simulink model "quad_6D0F_ASMC"  (R2023a)
settings: Solver=ode1  StartTime=0.0  StopTime=10.0  FixedStep=0.01  RelTol=1e-3
libraries: matrix_library x1, robotcorelib x1
settings Model: Creator=Adan Daniel  LastModifiedBy=Adan Daniel

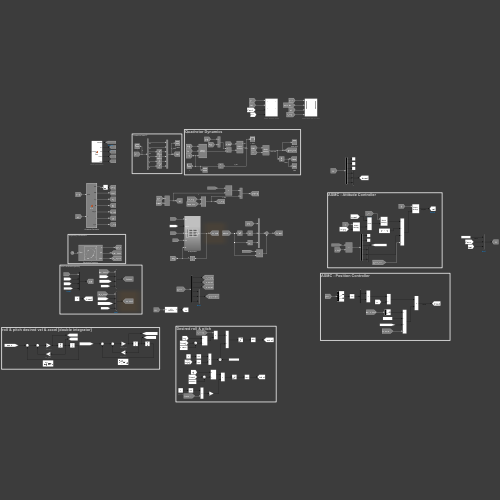
[thumbnail: Simulink's stored preview of the top-level diagram]
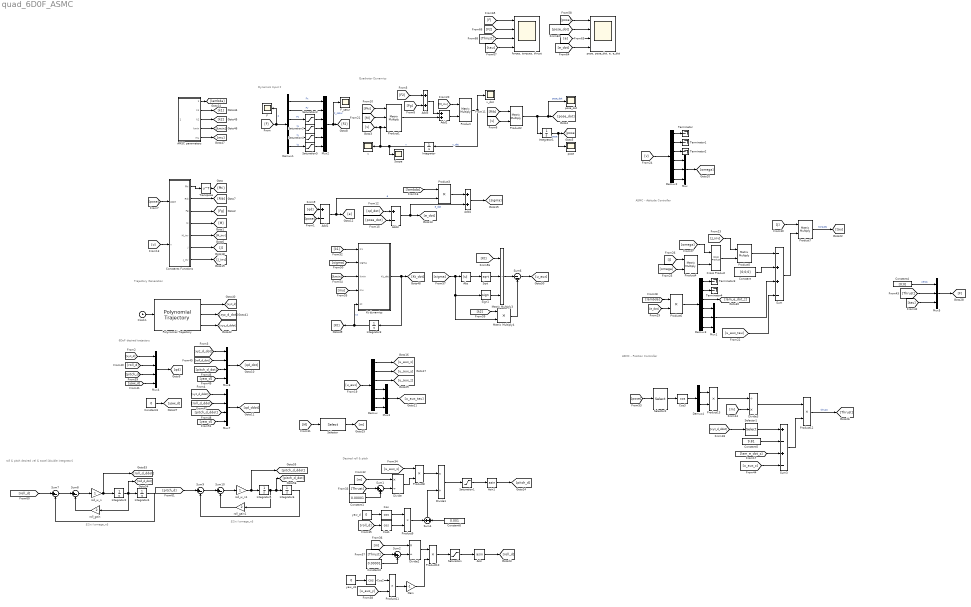
== system quad_6D0F_ASMC ==
  note: roll & pitch desired vel & accel [double integrator]
  note: Desired roll & pitch
  note: ASMC - Attitude Controller
  note: Quadrotor Dynamics
  note: Trajectory Generation
  note: Dynamics Input F
  note: $2\xi \omega_n$
  note: $2\xi \omega_n$
  note: 6DoF desired trajectory
  note: ASMC - Position Controller
  AMSC parameters : MATLAB Function  TreatAsAtomicUnit=on
  Abs : Abs  SaturateOnIntegerOverflow=off
  Add1 : Sum  Inputs=+-
  Add2 : Sum
  Add3 : Sum  Inputs=+-
  Add4 : Sum
  Add5 : Sum
  Asin : Trigonometry  Operator=asin
  Asin1 : Trigonometry  Operator=asin
  Clock1 : Clock
  Constant : Constant  Value=[0;0;0]
  Constant1 : Constant  Value=0.00001
  Constant2 : Constant  Value=0.00001
  Constant3 : Constant  Value=0
  Constant4 : Constant  Value=[0;0]
  Constant5 : Constant  Value=9.81
  Constant6 : Constant  Value=0.001
  Constants Functions : MATLAB Function  TreatAsAtomicUnit=on
  Cos{,1..3} (4 alike) : Trigonometry  Operator=cos
  Cross Product : matrix_library/Cross Product
  Demux{,1..3} (4 alike) : Demux  Outputs=6
  Demux4 : Demux  Outputs=2
  Divide : Product  Inputs=*/
  Divide1 : Product  Inputs=*/
  Divide2 : Product  Inputs=*/
  Divide3 : Product  Inputs=/*
  F : Scope
  F_satur : Scope
  Gain : Gain  Gain=-1
  Integrator : Integrator  InitialCondition=[0; 0; 0; 0; 0; 0]
  Integrator1 : Integrator  InitialCondition=[0; 0; 0; 0; 0; 0]
  Integrator{2,4..6} (4 alike) : Integrator
  Integrator3 : Integrator  InitialCondition=[0; 0; 0; 0; 0; 0]
  Kt dynamics : Subsystem
  Matrix Multiply3 : Product  Inputs=3
  Matrix Multiply4 : Product
  Mux{,1,3,5} (4 alike) : Mux  Inputs=3
  Mux2 : Mux  Inputs=6
  Mux4 : Mux
  Mux6 : Mux
  Mux7 : Mux
  Polynomial Trajectory : robotcorelib/Polynomial Trajectory  WaypointSource=Internal  Waypoints=[0, 0, 0, 0, 0, 0; 0, 0, 0, 0, 0, 0; 0, 0, 0, 0, 0, 0]  TimePoints=[ 0, 12, 24, 35, 48, 60]  TimeInterval=[ 1, 4 ]  Method=Cubic Polynomial  ParameterSource=Internal  VelocityBoundaryCondition=zeros( 3, 6)  AccelerationBoundaryCondition=zeros( 2, 5 )  SimulateUsing=Interpreted execution
  Product{,2,4..5,7} (5 alike) : Product  Multiplication=Matrix(*)
  Product1 : Product  Inputs=3  Multiplication=Matrix(*)
  Product{3,6,8..13} (8 alike) : Product
  Saturation : Saturate  UpperLimit=1  LowerLimit=-1
  Saturation1 : Saturate  UpperLimit=1  LowerLimit=-1
  Saturation2 : Saturate  UpperLimit=5.8*6  LowerLimit=0
  Saturation3 : Saturate
  Saturation4 : Saturate
  Saturation5 : Saturate
  Scope : Scope
  Selector : Selector  NumberOfDimensions=2  InputPortWidth=3  IndexOptions=Index vector (dialog),Index vector (dialog)  Indices=1,1  OutputSizes=1,1
  Selector1 : Selector  InputPortWidth=3  IndexOptions=Index vector (dialog)  Indices=3  OutputSizes=1
  Selector2 : Selector  InputPortWidth=6  IndexOptions=Index vector (dialog)  Indices=[4 5]  OutputSizes=1
  Sign1 : Signum
  Sqrt : Sqrt
  Sum : Sum  Inputs=-++-
  Sum1 : Sum  Inputs=|++
  Sum{7..10} (4 alike) : Sum  Inputs=|+-
  Sum2 : Sum  Inputs=|++
  Sum3 : Sum  Inputs=+-+-
  Sum4 : Sum
  Sum6 : Sum  Inputs=|--
  Terminator{,1..4} (5 alike) : Terminator
  Transpose : Math  Operator=transpose
  "forces, torques, thrust" : Scope  NumInputPorts=4
  pose : Scope
  "pose, pose_dot, e, e_dot" : Scope  NumInputPorts=4
  pose_dot : Scope
  roll_gain : Gain  Gain=2
  roll_gain1 : Gain  Gain=2
  roll_w_n : Gain
  roll_w_n1 : Gain
  v : Scope
  v_dot : Scope
  yaw_d : Constant  Value=0
  yaw_d1 : Constant  Value=0
  wires:
  [v] -> Product2/2
  Product2/1 -> Integrator1/1, pose_dot/1, [pose_dot]  "pose_dot"
  Product/1 -> v_dot/1, Integrator/1  "v_dot"
  Integrator1/1 -> pose/1, [pose]  "pose"
  Integrator/1 -> Scope/1, v/1, [v], Product1/3  "v"
  Add5/1 -> Add2/1
  [M] -> Product1/2
  [Fg] -> Add5/2
  Add2/1 -> Product/2
  [Rib] -> Product2/1
  [Phi] -> Product1/1
  Product1/1 -> Add2/2
  [F2] -> Add5/1
  [M_inv] -> Product/1
  [pose] -> Constants Functions/1(pose)
  [v] -> Constants Functions/2(v)
  Constants Functions/1(Phi) -> Transpose/1
  Constants Functions/4(M) -> [M]
  Constants Functions/3(Fg) -> [Fg]
  Constants Functions/5(M_inv) -> [M_inv]
  Constants Functions/2(Rib) -> [Rib]
  Transpose/1 -> [Phi]
  Clock1/1 -> Polynomial Trajectory/1
  Saturation5/1 -> Mux2/6
  Demux1/5 -> Saturation4/1  "ty"
  Saturation3/1 -> Mux2/4
  Saturation2/1 -> Mux2/3
  Demux1/1 -> Mux2/1  "Fx"
  Demux1/2 -> Mux2/2  "Fy"
  Mux2/1 -> F_satur/1, [F2]  "F_satur"
  [F] -> F/1, Demux1/1  "F"
  Saturation4/1 -> Mux2/5
  Demux1/6 -> Saturation5/1  "tz"
  Demux1/4 -> Saturation3/1  "tx"
  Demux1/3 -> Saturation2/1  "Fz"
  AMSC parameters/5(mu) -> [mu]
  AMSC parameters/2(k1) -> [k1]
  AMSC parameters/3(k2) -> [k2]
  AMSC parameters/4(kmin) -> [kmin]
  Polynomial Trajectory/1 -> [xyz_d]
  Polynomial Trajectory/2 -> [xyz_d_dot]
  Polynomial Trajectory/3 -> [xyz_d_ddot]
  [qd] -> Add1/1
  [pose] -> Add1/2
  [qd_dot] -> Add3/1
  AMSC parameters/1(lambda) -> [lambda]
  [lambda] -> Product3/1
  Add1/1 -> Product3/2, [e]  "e"
  Product3/1 -> Add4/1
  Add3/1 -> Add4/2, [e_dot]  "e_dot"
  Add4/1 -> [sigma]
  Abs/1 -> Sqrt/1
  Integrator3/1 -> [Kt], Kt dynamics/5(Kt)  "Kt"
  [sigma] -> Matrix Multiply4/2, Sign1/1, Abs/1
  Sign1/1 -> Matrix Multiply3/3
  Matrix Multiply4/1 -> Sum6/2
  [mu] -> Kt dynamics/4(mu)
  Sqrt/1 -> Matrix Multiply3/2
  [k2] -> Matrix Multiply4/1
  [sigma] -> Kt dynamics/2(sigma)
  [k1] -> Kt dynamics/1(K1)
  [Kt] -> Matrix Multiply3/1
  [kmin] -> Kt dynamics/3(Kmin)
  Matrix Multiply3/1 -> Sum6/1
  Kt dynamics/1(Kt_dot) -> Integrator3/1, [Kt_dot]
  Sum6/1 -> [u_aux]
  [u_aux] -> Demux/1
  Demux/1 -> [u_aux_x]
  Demux/2 -> [u_aux_y]
  Constants Functions/7(J_inv) -> [J_inv]
  Constants Functions/6(J) -> [J]
  [v] -> Demux2/1
  Demux2/4 -> Mux/1
  Demux2/6 -> Mux/3
  Demux2/5 -> Mux/2
  Mux/1 -> [omega]
  [J] -> Product4/1
  [omega] -> Product4/2
  Product4/1 -> Cross Product/2
  [omega] -> Cross Product/1
  Cross Product/1 -> Product5/2
  [J_inv] -> Product5/1
  [lambda] -> Product6/1
  [e_dot] -> Product6/2
  Mux1/1 -> Sum/3
  Demux3/4 -> Mux1/1
  Demux3/6 -> Mux1/3
  Demux3/5 -> Mux1/2
  Product6/1 -> Demux3/1
  Mux3/1 -> [u_aux_tau]
  Demux/4 -> Mux3/1
  Demux/6 -> Mux3/3
  Demux/5 -> Mux3/2
  Product5/1 -> Sum/1
  Constant/1 -> Sum/2
  [u_aux_tau] -> Sum/4
  [J] -> Product7/1
  Sum/1 -> Product7/2
  Product7/1 -> [tau]  "torques"
  [M] -> Selector/1
  Selector/1 -> [m]
  [pose_dot] -> Add3/2
  Constant3/1 -> [yaw_d]
  [yaw_d] -> Mux4/4
  [pitch_d] -> Mux4/3
  [roll_d] -> Mux4/2
  [xyz_d] -> Mux4/1
  Mux4/1 -> [qd]
  Demux2/1 -> Terminator/1
  Demux2/2 -> Terminator1/1
  Demux2/3 -> Terminator2/1
  Demux3/2 -> Terminator4/1
  Demux3/1 -> Terminator3/1
  Demux3/3 -> [lam_e_dot_z]
  Constant4/1 -> Mux5/1  "zeros"
  [Thrust] -> Mux5/2
  [tau] -> Mux5/3
  Mux5/1 -> [F]
  Demux/3 -> [u_aux_z]
  Divide1/1 -> Saturation1/1
  [u_aux_y] -> Product11/2
  Cos1/1 -> Product9/2
  [m] -> Divide2/1
  Sum1/1 -> Divide/2
  Gain/1 -> Product10/2
  [Thrust] -> Sum2/1
  yaw_d1/1 -> Cos2/1
  Constant1/1 -> Sum1/2
  Product11/1 -> Gain/1
  Cos/1 -> Product9/1
  Product10/1 -> Saturation/1
  Constant2/1 -> Sum2/2
  [roll_d] -> Cos1/1
  Divide2/1 -> Product10/1
  Divide/1 -> Product8/2
  Sum2/1 -> Divide2/2
  [u_aux_x] -> Product8/1
  Cos2/1 -> Product11/1
  Asin1/1 -> [pitch_d]
  [Thrust] -> Sum1/1
  Saturation/1 -> Asin/1
  Saturation1/1 -> Asin1/1
  yaw_d/1 -> Cos/1
  Product8/1 -> Divide1/1
  [m] -> Divide/1
  Asin/1 -> [roll_d]
  Sum7/1 -> Sum8/1
  [roll_d] -> Sum7/1
  Integrator2/1 -> [roll_d_dot], Integrator4/1, roll_gain/1
  roll_gain/1 -> Sum8/2
  Integrator6/1 -> Sum9/2
  Sum9/1 -> Sum10/1
  Sum8/1 -> roll_w_n/1
  Integrator4/1 -> Sum7/2
  Integrator5/1 -> roll_gain1/1, [pitch_d_dot], Integrator6/1
  roll_w_n/1 -> [roll_d_ddot], Integrator2/1
  roll_w_n1/1 -> [pitch_d_ddot], Integrator5/1
  roll_gain1/1 -> Sum10/2
  [pitch_d] -> Sum9/1
  Sum10/1 -> roll_w_n1/1
  [yaw_d] -> Mux6/4
  [roll_d_dot] -> Mux6/2
  [xyz_d_dot] -> Mux6/1
  [pitch_d_dot] -> Mux6/3
  Mux6/1 -> [qd_dot]
  [yaw_d] -> Mux7/4
  [roll_d_ddot] -> Mux7/2
  [xyz_d_ddot] -> Mux7/1
  [pitch_d_ddot] -> Mux7/3
  Mux7/1 -> [qd_ddot]
  [u_aux_z] -> Sum3/4
  [lam_e_dot_z] -> Sum3/3
  Constant5/1 -> Sum3/2
  Selector1/1 -> Sum3/1
  [xyz_d_ddot] -> Selector1/1
  [pose] -> Selector2/1
  Selector2/1 -> Cos3/1
  Cos3/1 -> Demux4/1
  Demux4/1 -> Product13/1
  Demux4/2 -> Product13/2
  [m] -> Divide3/2
  Sum3/1 -> Product12/2
  Divide3/1 -> Product12/1
  Product13/1 -> Divide3/1
  Product12/1 -> [Thrust]  "thrust"
  [pose] -> "pose, pose_dot, e, e_dot"/1
  [e_dot] -> "pose, pose_dot, e, e_dot"/4
  [e] -> "pose, pose_dot, e, e_dot"/3
  [pose_dot] -> "pose, pose_dot, e, e_dot"/2
  [tau] -> "forces, torques, thrust"/4
  [F2] -> "forces, torques, thrust"/2
  [F] -> "forces, torques, thrust"/1
  [Thrust] -> "forces, torques, thrust"/3
  Product9/1 -> Sum4/1
  Sum4/1 -> Divide1/2
  Constant6/1 -> Sum4/2

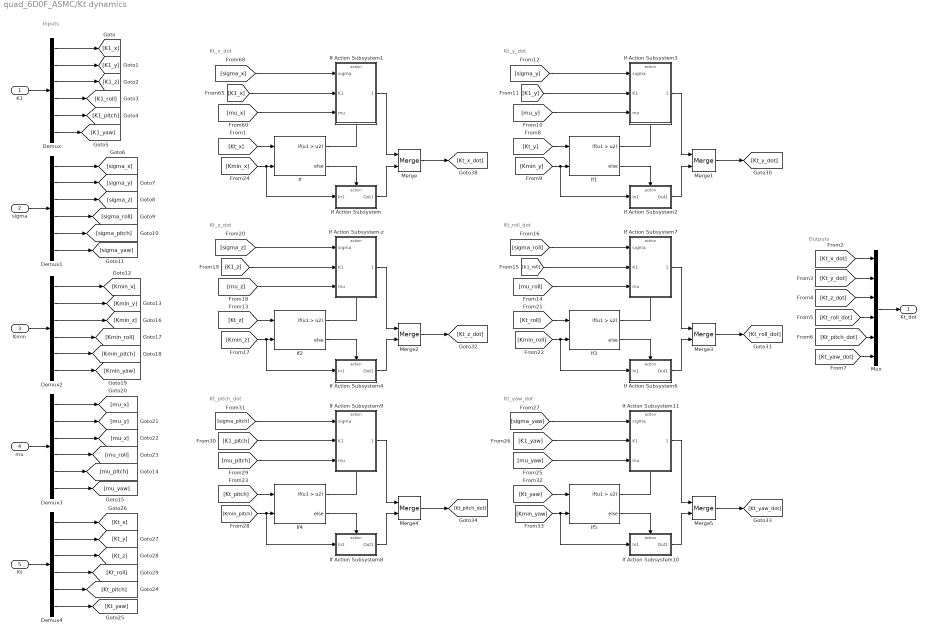
== system quad_6D0F_ASMC/Kt dynamics ==
  note: Outputs
  note: Inputs
  note: Kt_x_dot
  note: Kt_y_dot
  note: Kt_z_dot
  note: Kt_roll_dot
  note: Kt_pitch_dot
  note: Kt_yaw_dot
  K1 : Inport
  sigma : Inport  Port=2
  Kmin : Inport  Port=3
  mu : Inport  Port=4
  Kt : Inport  Port=5
  Demux{,1..4} (5 alike) : Demux  Outputs=6
  If{,1..5} (6 alike) : If  NumInputs=2  IfExpression=u1 > u2
  If Action Subsystem : Subsystem  TreatAsAtomicUnit=on
  If Action Subsystem-z : Subsystem  TreatAsAtomicUnit=on
  If Action Subsystem1 : Subsystem  TreatAsAtomicUnit=on
  If Action Subsystem10 : Subsystem  TreatAsAtomicUnit=on
  If Action Subsystem11 : Subsystem  TreatAsAtomicUnit=on
  If Action Subsystem2 : Subsystem  TreatAsAtomicUnit=on
  If Action Subsystem3 : Subsystem  TreatAsAtomicUnit=on
  If Action Subsystem4 : Subsystem  TreatAsAtomicUnit=on
  If Action Subsystem6 : Subsystem  TreatAsAtomicUnit=on
  If Action Subsystem7 : Subsystem  TreatAsAtomicUnit=on
  If Action Subsystem8 : Subsystem  TreatAsAtomicUnit=on
  If Action Subsystem9 : Subsystem  TreatAsAtomicUnit=on
  Merge{,1..5} (6 alike) : Merge
  Mux : Mux  Inputs=6
  Kt_dot : Outport
  wires:
  [Kt_x] -> If/1
  [sigma_x] -> If Action Subsystem1/1(sigma)
  If/1 -> If Action Subsystem1/Action
  [K1_x] -> If Action Subsystem1/2(K1)
  If Action Subsystem1/1(Kt_x_dot) -> Merge/1
  If Action Subsystem/1(Out1) -> Merge/2
  If/2 -> If Action Subsystem/Action
  Merge/1 -> [Kt_x_dot]
  [Kmin_x] -> If Action Subsystem/1(In1), If/2
  [mu_x] -> If Action Subsystem1/3(mu)
  Merge1/1 -> [Kt_y_dot]
  If1/2 -> If Action Subsystem2/Action
  If Action Subsystem2/1(Out1) -> Merge1/2
  If Action Subsystem3/1(Kt_x_dot) -> Merge1/1
  [Kt_y] -> If1/1
  [K1_y] -> If Action Subsystem3/2(K1)
  [mu_y] -> If Action Subsystem3/3(mu)
  [Kmin_y] -> If Action Subsystem2/1(In1), If1/2
  [sigma_y] -> If Action Subsystem3/1(sigma)
  Merge2/1 -> [Kt_z_dot]
  If Action Subsystem-z/1(Kt_z_dot) -> Merge2/1
  [sigma_z] -> If Action Subsystem-z/1(sigma)
  [Kt_z] -> If2/1
  [mu_z] -> If Action Subsystem-z/3(mu)
  [Kmin_z] -> If Action Subsystem4/1(In1), If2/2
  If3/2 -> If Action Subsystem6/Action
  If Action Subsystem7/1(Kt_x_dot) -> Merge3/1
  Merge3/1 -> [Kt_roll_dot]
  If3/1 -> If Action Subsystem7/Action
  [Kmin_roll] -> If Action Subsystem6/1(In1), If3/2
  If2/2 -> If Action Subsystem4/Action
  [sigma_roll] -> If Action Subsystem7/1(sigma)
  If2/1 -> If Action Subsystem-z/Action
  [K1_roll] -> If Action Subsystem7/2(K1)
  If Action Subsystem6/1(Out1) -> Merge3/2
  [mu_roll] -> If Action Subsystem7/3(mu)
  If Action Subsystem4/1(Out1) -> Merge2/2
  [Kt_roll] -> If3/1
  [K1_z] -> If Action Subsystem-z/2(K1)
  Merge4/1 -> [Kt_pitch_dot]
  If Action Subsystem9/1(Kt_x_dot) -> Merge4/1
  [sigma_pitch] -> If Action Subsystem9/1(sigma)
  [Kt_pitch] -> If4/1
  [mu_pitch] -> If Action Subsystem9/3(mu)
  [Kmin_pitch] -> If Action Subsystem8/1(In1), If4/2
  If5/2 -> If Action Subsystem10/Action
  If Action Subsystem11/1(Kt_x_dot) -> Merge5/1
  Merge5/1 -> [Kt_yaw_dot]
  If5/1 -> If Action Subsystem11/Action
  [Kmin_yaw] -> If Action Subsystem10/1(In1), If5/2
  If4/2 -> If Action Subsystem8/Action
  [sigma_yaw] -> If Action Subsystem11/1(sigma)
  If4/1 -> If Action Subsystem9/Action
  [K1_yaw] -> If Action Subsystem11/2(K1)
  If Action Subsystem10/1(Out1) -> Merge5/2
  [mu_yaw] -> If Action Subsystem11/3(mu)
  If Action Subsystem8/1(Out1) -> Merge4/2
  [Kt_yaw] -> If5/1
  [K1_pitch] -> If Action Subsystem9/2(K1)
  If1/1 -> If Action Subsystem3/Action
  Demux4/6 -> [Kt_yaw]
  Demux4/1 -> [Kt_x]
  Demux1/5 -> [sigma_pitch]
  Demux1/3 -> [sigma_z]
  Demux1/1 -> [sigma_x]
  Demux1/2 -> [sigma_y]
  Kt/1 -> Demux4/1
  Demux4/4 -> [Kt_roll]
  sigma/1 -> Demux1/1
  Demux3/4 -> [mu_roll]
  Demux2/4 -> [Kmin_roll]
  Demux3/1 -> [mu_x]
  Demux2/3 -> [Kmin_z]
  Demux3/3 -> [mu_z]
  mu/1 -> Demux3/1
  Demux3/6 -> [mu_yaw]
  Demux3/5 -> [mu_pitch]
  Demux2/5 -> [Kmin_pitch]
  Demux3/2 -> [mu_y]
  Demux2/6 -> [Kmin_yaw]
  Demux2/1 -> [Kmin_x]
  Demux2/2 -> [Kmin_y]
  Demux/4 -> [K1_roll]
  Demux1/4 -> [sigma_roll]
  Demux4/5 -> [Kt_pitch]
  Demux4/2 -> [Kt_y]
  Demux4/3 -> [Kt_z]
  Demux/1 -> [K1_x]
  K1/1 -> Demux/1
  Demux/6 -> [K1_yaw]
  Demux/5 -> [K1_pitch]
  Demux1/6 -> [sigma_yaw]
  Demux/2 -> [K1_y]
  Kmin/1 -> Demux2/1
  Demux/3 -> [K1_z]
  Mux/1 -> Kt_dot/1
  [Kt_z_dot] -> Mux/3
  [Kt_yaw_dot] -> Mux/6
  [Kt_pitch_dot] -> Mux/5
  [Kt_x_dot] -> Mux/1
  [Kt_y_dot] -> Mux/2
  [Kt_roll_dot] -> Mux/4

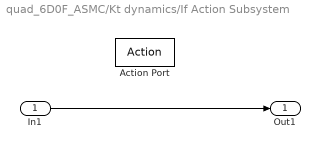
== system quad_6D0F_ASMC/Kt dynamics/If Action Subsystem ==
  In1 : Inport
  Action Port : ActionPort  ActionPortLabel=else
  Out1 : Outport
  wires:
  In1/1 -> Out1/1

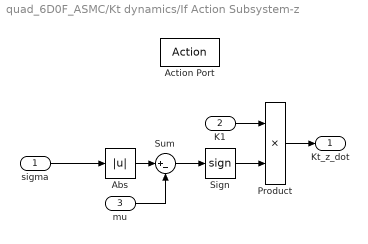
== system quad_6D0F_ASMC/Kt dynamics/If Action Subsystem-z ==
  sigma : Inport
  K1 : Inport  Port=2
  mu : Inport  Port=3
  Action Port : ActionPort  ActionPortLabel=if(u1 > u2)
  Abs : Abs  SaturateOnIntegerOverflow=off
  Product : Product
  Sign : Signum
  Sum : Sum  Inputs=|+-
  Kt_z_dot : Outport
  wires:
  sigma/1 -> Abs/1
  Abs/1 -> Sum/1
  mu/1 -> Sum/2
  Sum/1 -> Sign/1
  Product/1 -> Kt_z_dot/1
  Sign/1 -> Product/2
  K1/1 -> Product/1

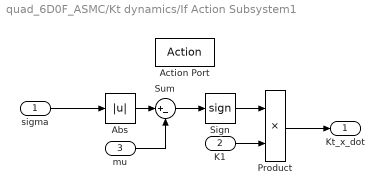
== system quad_6D0F_ASMC/Kt dynamics/If Action Subsystem1 ==
  sigma : Inport
  K1 : Inport  Port=2
  mu : Inport  Port=3
  Action Port : ActionPort  ActionPortLabel=if(u1 > u2)
  Abs : Abs  SaturateOnIntegerOverflow=off
  Product : Product
  Sign : Signum
  Sum : Sum  Inputs=|+-
  Kt_x_dot : Outport
  wires:
  sigma/1 -> Abs/1
  Abs/1 -> Sum/1
  mu/1 -> Sum/2
  Sum/1 -> Sign/1
  Sign/1 -> Product/1
  K1/1 -> Product/2
  Product/1 -> Kt_x_dot/1

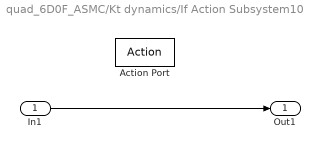
== system quad_6D0F_ASMC/Kt dynamics/If Action Subsystem10 ==
  In1 : Inport
  Action Port : ActionPort  ActionPortLabel=else
  Out1 : Outport
  wires:
  In1/1 -> Out1/1

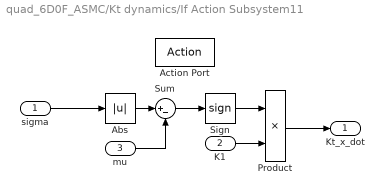
== system quad_6D0F_ASMC/Kt dynamics/If Action Subsystem11 ==
  sigma : Inport
  K1 : Inport  Port=2
  mu : Inport  Port=3
  Action Port : ActionPort  ActionPortLabel=if(u1 > u2)
  Abs : Abs  SaturateOnIntegerOverflow=off
  Product : Product
  Sign : Signum
  Sum : Sum  Inputs=|+-
  Kt_x_dot : Outport
  wires:
  sigma/1 -> Abs/1
  Abs/1 -> Sum/1
  mu/1 -> Sum/2
  Sum/1 -> Sign/1
  Sign/1 -> Product/1
  K1/1 -> Product/2
  Product/1 -> Kt_x_dot/1

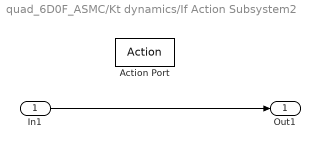
== system quad_6D0F_ASMC/Kt dynamics/If Action Subsystem2 ==
  In1 : Inport
  Action Port : ActionPort  ActionPortLabel=else
  Out1 : Outport
  wires:
  In1/1 -> Out1/1

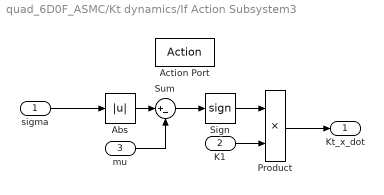
== system quad_6D0F_ASMC/Kt dynamics/If Action Subsystem3 ==
  sigma : Inport
  K1 : Inport  Port=2
  mu : Inport  Port=3
  Action Port : ActionPort  ActionPortLabel=if(u1 > u2)
  Abs : Abs  SaturateOnIntegerOverflow=off
  Product : Product
  Sign : Signum
  Sum : Sum  Inputs=|+-
  Kt_x_dot : Outport
  wires:
  sigma/1 -> Abs/1
  Abs/1 -> Sum/1
  mu/1 -> Sum/2
  Sum/1 -> Sign/1
  Sign/1 -> Product/1
  K1/1 -> Product/2
  Product/1 -> Kt_x_dot/1

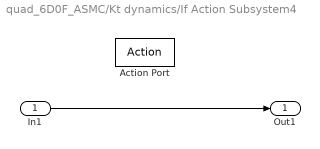
== system quad_6D0F_ASMC/Kt dynamics/If Action Subsystem4 ==
  In1 : Inport
  Action Port : ActionPort  ActionPortLabel=else
  Out1 : Outport
  wires:
  In1/1 -> Out1/1

== system quad_6D0F_ASMC/Kt dynamics/If Action Subsystem6 ==
  In1 : Inport
  Action Port : ActionPort  ActionPortLabel=else
  Out1 : Outport
  wires:
  In1/1 -> Out1/1

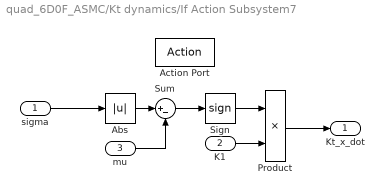
== system quad_6D0F_ASMC/Kt dynamics/If Action Subsystem7 ==
  sigma : Inport
  K1 : Inport  Port=2
  mu : Inport  Port=3
  Action Port : ActionPort  ActionPortLabel=if(u1 > u2)
  Abs : Abs  SaturateOnIntegerOverflow=off
  Product : Product
  Sign : Signum
  Sum : Sum  Inputs=|+-
  Kt_x_dot : Outport
  wires:
  sigma/1 -> Abs/1
  Abs/1 -> Sum/1
  mu/1 -> Sum/2
  Sum/1 -> Sign/1
  Sign/1 -> Product/1
  K1/1 -> Product/2
  Product/1 -> Kt_x_dot/1

== system quad_6D0F_ASMC/Kt dynamics/If Action Subsystem8 ==
  In1 : Inport
  Action Port : ActionPort  ActionPortLabel=else
  Out1 : Outport
  wires:
  In1/1 -> Out1/1

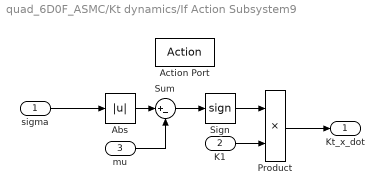
== system quad_6D0F_ASMC/Kt dynamics/If Action Subsystem9 ==
  sigma : Inport
  K1 : Inport  Port=2
  mu : Inport  Port=3
  Action Port : ActionPort  ActionPortLabel=if(u1 > u2)
  Abs : Abs  SaturateOnIntegerOverflow=off
  Product : Product
  Sign : Signum
  Sum : Sum  Inputs=|+-
  Kt_x_dot : Outport
  wires:
  sigma/1 -> Abs/1
  Abs/1 -> Sum/1
  mu/1 -> Sum/2
  Sum/1 -> Sign/1
  Sign/1 -> Product/1
  K1/1 -> Product/2
  Product/1 -> Kt_x_dot/1

== matlab function quad_6D0F_ASMC/AMSC parameters ==
  data: lambda output; unused input; k1 output; k2 output; kmin output; mu output
function [lambda, k1, k2, kmin, mu]= fcn(~)

lambda = [1; 1; 1; 1; 1; 1];

k1 = [1; 1; 1; 1; 1; 1];

k2 = [1; 1; 1; 1; 1; 1];

kmin = [1; 1; 1; 1; 1; 1];

mu = [0.01; 0.01; 0.01; 0.01; 0.01; 0.01];

== matlab function quad_6D0F_ASMC/Constants Functions ==
  data: Phi output; Rib output; Fg output; pose input; M output; M_inv output; v input; J output; J_inv output
function [Phi, Rib, Fg, M, M_inv, J, J_inv]   = fcn(pose, v)

%% System constants
m = 2; %5 mass 2.2 kg
l = 0.25; % m
g = 9.81; % gravity
Jxx =  0.0411; % kg m²
Jyy = 0.0478; % kg m²
Jzz = 0.0599; % kg m²
kT = 3.4e-5;
kQ = 3.4e-6;
%% Phi vector 6d

uu = v(1);
vv = v(2);
ww = v(3);
pp = v(4);
qq = v(5);
rr = v(6);


Phi = [0, -rr, qq, 0, -ww, vv;
        rr, 0, -pp , ww, 0, -uu;
        -qq, pp, 0,  -vv, uu, 0;
        0, 0, 0, 0, -rr, qq; 
        0, 0, 0, rr, 0, -pp;
        0, 0, 0, -qq, pp, 0];
%% Fg and Rib calculation

roll = pose(4);
pitch = pose(5);
yaw = pose(6);


Rib = [cos(yaw)*cos(pitch), -cos(roll)*sin(yaw) + cos(yaw)*sin(roll)*sin(pitch), sin(roll)*sin(yaw) + cos(roll)*cos(yaw)*sin(pitch), 0, 0, 0;
       cos(pitch)*sin(yaw), cos(roll)*cos(yaw) + sin(yaw)*sin(pitch)*sin(roll), -cos(yaw)*sin(roll) + sin(yaw)*sin(pitch)*cos(roll), 0, 0, 0;
       -sin(pitch), cos(pitch)*sin(roll), cos(pitch)*cos(roll), 0, 0, 0;
       0, 0, 0, 1, sin(roll)*tan(pitch), cos(roll)*tan(pitch);
       0, 0, 0, 0, cos(roll), -sin(roll);
       0, 0, 0, 0, sin(roll)/cos(pitch), cos(roll)/cos(pitch)];

Fg = [m*g*sin(pitch);
      -m*g*cos(pitch)*sin(roll);
      -m*g*cos(pitch)*cos(roll);
      0;
      0;
      0];

%% M matrix

M = [m, 0, 0, 0, 0, 0;
    0, m, 0, 0, 0, 0;
    0, 0, m, 0, 0, 0;
    0, 0, 0, Jxx, 0, 0;
    0, 0, 0, 0, Jyy, 0;
    0, 0, 0, 0, 0, Jzz];

M_inv = inv(M);

%% Allocation matrix

% allo = [0, 0, 0, 0, 0, 0;
%         0, 0, 0, 0, 0, 0;
%         kT, kT, kT, kT, kT, kT;
%         -kT*l, kT*l, kT*l/2, -kT*l/2, -kT*l/2, kT*l/2;
%         0, 0, -sqrt(3)*kT*l/2, sqrt(3)*kT*l/2, -sqrt(3)*kT*l/2, sqrt(3)*kT*l/2;
%         kQ, -kQ, kQ, -kQ, -kQ, kQ,];
% 
% allo = pinv(allo);

J = [Jxx, 0, 0;
     0, Jyy, 0;
     0, 0, Jzz];

J_inv = inv(J);
